simulink model "Final_Cloud"  (R2026a)
settings: Solver=FixedStepAuto  StopTime=inf  FixedStep=0.01  EnableMultiTasking=on
undefined symbols (not defined in the file or in its folder): Kg, Kt, r, R_m, V_batt
libraries: arduinolib x7, arduinosensorlib x1, slpidlib x1
settings Model: SimulationMode=external  SILPILModeSetting=veronly  ExtModeTrigDuration=2  Creator=Adham  LastModifiedBy=Adham
settings HardwareCC: ProdLargestAtomicInteger=Long  ProdLargestAtomicFloat=Double  ProdHWDeviceType=ARM Compatible->ARM Cortex  UseEmbeddedCoderFeatures=off
settings RTWCC: SystemTargetFile=ert.tlc  HardwareBoard=ESP32-WROOM (Arduino Compatible)  TLCOptions="-aInlineSetEventsForThisBaseRateFcn=TLC_FALSE -aSuppressMultiTaskScheduler=TLC_FALSE  -aRateBasedStepFcn=0"  Toolchain=ESP32  BuildConfiguration=Faster Runs  Description=Embedded Coder
settings RTWCC: CustomInclude=|
  | C:\ProgramData\MATLAB\SupportPackages\R2026a\aCLI\data\packages\esp32\hardware\esp32\2.0.17\libraries\Wire\src
  | D:\CoTune2026\Active_Suspension_resources\Parameter_Estimation_DAQ
  | D:\CoTune2026\Active_Suspension_resources\Parameter_Estimation_DAQ\core\inc
  | D:\CoTune2026\Active_Suspension_resources\Parameter_Estimation_DAQ\core\src
  | D:\CoTune2026\Active_Suspension_resources\Parameter_Estimation_DAQ\platform\inc
  | D:\CoTune2026\Active_Suspension_resources\Parameter_Estimation_DAQ\platform\src
  | C:\ProgramData\MATLAB\SupportPackages\R2026a\aCLI\data\packages\esp32\hardware\esp32\2.0.17\libraries\WiFi\src
  | C:\ProgramData\MATLAB\SupportPackages\R2026a\aCLI\data\packages\esp32\hardware\esp32\2.0.17\libraries\WiFiClientSecure\src
  | C:\Users\Dell\Documents\Arduino\libraries\PubSubClient\src
  | C:\Users\Dell\Documents\Arduino\libraries\ArduinoJson\src
settings RTWCC: CustomSource=|
  | C:\ProgramData\MATLAB\SupportPackages\R2026a\aCLI\data\packages\esp32\hardware\esp32\2.0.17\libraries\Wire\src\Wire.cpp
  | core\src\vl53l0x_api.cpp
  | core\src\vl53l0x_api_calibration.cpp
  | core\src\vl53l0x_api_core.cpp
  | core\src\vl53l0x_api_ranging.cpp
  | core\src\vl53l0x_api_strings.cpp
  | platform\src\vl53l0x_platform.cpp
  | Adafruit_VL53L0X.cpp
  | C:\Users\Dell\Documents\Arduino\libraries\PubSubClient\src\PubSubClient.cpp
  | C:\ProgramData\MATLAB\SupportPackages\R2026a\aCLI\data\packages\esp32\hardware\esp32\2.0.17\libraries\WiFi\src\WiFi.cpp
  | C:\ProgramData\MATLAB\SupportPackages\R2026a\aCLI\data\packages\esp32\hardware\esp32\2.0.17\libraries\WiFi\src\WiFiSTA.cpp
  | C:\ProgramData\MATLAB\SupportPackages\R2026a\aCLI\data\packages\esp32\hardware\esp32\2.0.17\libraries\WiFi\src\WiFiGeneric.cpp
  | C:\ProgramData\MATLAB\SupportPackages\R2026a\aCLI\data\packages\esp32\hardware\esp32\2.0.17\libraries\WiFi\src\WiFiClient.cpp
  | C:\ProgramData\MATLAB\SupportPackages\R2026a\aCLI\data\packages\esp32\hardware\esp32\2.0.17\libraries\WiFiClientSecure\src\WiFiClientSecure.cpp
  | C:\ProgramData\MATLAB\SupportPackages\R2026a\aCLI\data\packages\esp32\hardware\esp32\2.0.17\libraries\WiFiClientSecure\src\ssl_client.cpp
  | C:\ProgramData\MATLAB\SupportPackages\R2026a\aCLI\data\packages\esp32\hardware\esp32\2.0.17\libraries\WiFi\src\WiFiScan.cpp
  | C:\ProgramData\MATLAB\SupportPackages\R2026a\aCLI\data\packages\esp32\hardware\esp32\2.0.17\libraries\WiFi\src\WiFiAP.cpp
  | C:\ProgramData\MATLAB\SupportPackages\R2026a\aCLI\data\packages\esp32\hardware\esp32\2.0.17\libraries\WiFi\src\WiFiUdp.cpp
settings ERTTargetCC: ExtModeTransport=3.0  ExtModeAutomaticAllocSize=off  ExtModeStaticAllocSize=65536.0  SupportContinuousTime=on  SupportNonInlinedSFcns=on  SupportVariableSizeSignals=on

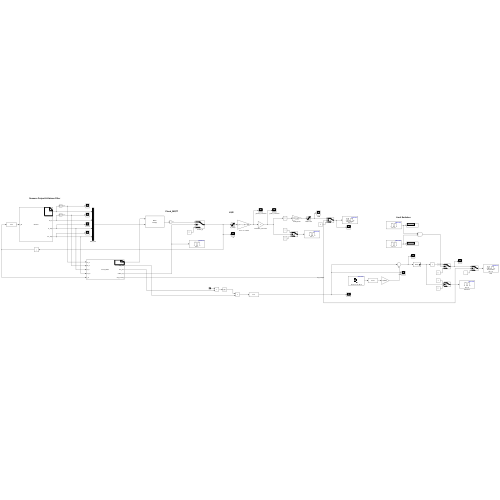
[thumbnail: Simulink's stored preview of the top-level diagram]
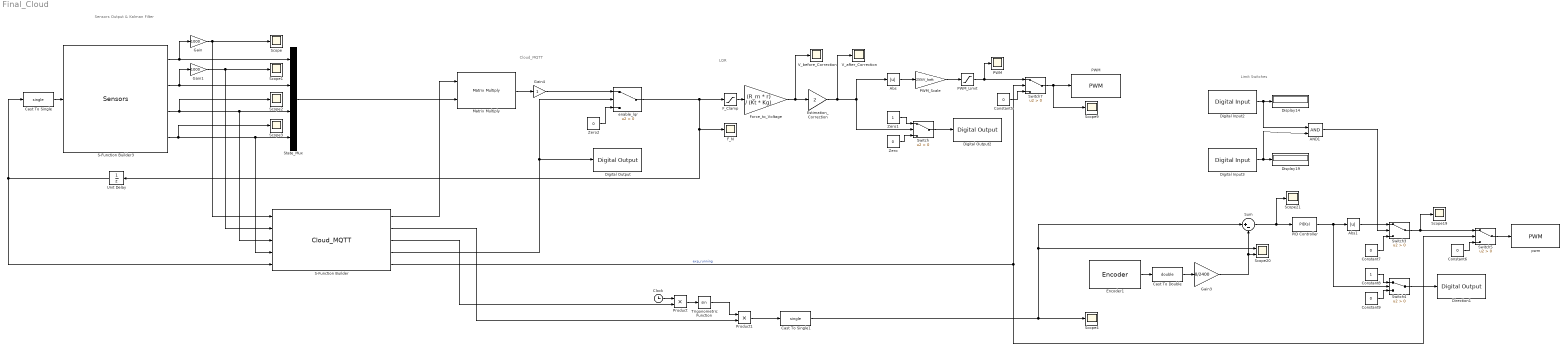
== system Final_Cloud ==
  note: Limit Switches
  note: Sensors Output & Kalman Filter
  note: LQR
  note: Cloud_MQTT
  AND1 : Logic  IconShape=distinctive  AllPortsSameDT=off  OutDataTypeStr=boolean
  Abs : Abs  SaturateOnIntegerOverflow=off
  Abs1 : Abs  SaturateOnIntegerOverflow=off
  Cast To Double : DataTypeConversion  OutDataTypeStr=double  SaturateOnIntegerOverflow=off  RndMeth=Floor
  Cast To Single : DataTypeConversion  OutDataTypeStr=single  SaturateOnIntegerOverflow=off  RndMeth=Floor
  Cast To Single1 : DataTypeConversion  OutDataTypeStr=single  SaturateOnIntegerOverflow=off  RndMeth=Floor
  Clock : Clock
  Constant{5..7,9} (4 alike) : Constant  Value=0
  Constant8 : Constant
  Digital Input2 : arduinolib/Digital Input  pinNumber=16  mode=Input Pullup  Direction=input  SampleTime=0.1  blockPlatform=arduino
  Digital Input3 : arduinolib/Digital Input  pinNumber=17  mode=Input Pullup  Direction=input  SampleTime=0.1  blockPlatform=arduino
  Digital Output : arduinolib/Digital Output  pinNumber=2  Direction=output  blockPlatform=arduino
  Digital Output2 : arduinolib/Digital Output  pinNumber=4  Direction=output  blockPlatform=arduino
  Direction1 : arduinolib/Digital Output  pinNumber=18  Direction=output  blockPlatform=arduino
  Display14 : Display
  Display19 : Display
  Encoder1 : arduinosensorlib/Encoder  InputA=13  InputB=14  Mode=No reset  SampleTime=-1
  Estimation_Correction : Gain  Gain=2
  F_Clamp : Saturate  UpperLimit=10  LowerLimit=-10
  F_N : Scope
      settings: ActiveDisplayYMinimum=-32.354349136352539  ActiveDisplayYMaximum=27.611242294311523  DataLoggingVariableName=ScopeData5
  Force_to_Voltage : Gain  Gain=(R_m * r) / (Kt * Kg)
  Gain : Gain  Gain=1000
  Gain1 : Gain  Gain=1000
  Gain3 : Gain  Gain=8/2400
  Gain4 : Gain
  Matrix Multiply : Product  Multiplication=Matrix(*)
  PID Controller : slpidlib/PID Controller  Controller=PID  Form=Parallel  TimeDomain=Continuous-time  UseExternalTs=off  SampleTime=-1  IntegratorMethod=Forward Euler  FilterMethod=Forward Euler  ControllerParametersSource=internal  P=20  I=0  UseKiTs=off  D=0  UseExternalDerivativeSource=off  N=100  UseFilter=on  TunerSelectOption=Transfer Function Based (PID Tuner App)  InitialConditionSource=internal  InitialConditionForIntegrator=0  InitialConditionForFilter=0  DifferentiatorICPrevScaledInput=0  ExternalReset=none  TrackingMode=off  Kt=1  LimitOutput=on  SatLimitsSource=internal  UpperSaturationLimit=255  LowerSaturationLimit=-255  LinearizeAsGain=on  AntiWindupMode=none  Kb=1  LimitIntegrator=off  UpperIntegratorSaturationLimit=inf  LowerIntegratorSaturationLimit=-inf  POutMin=[]  POutMax=[]  IOutMin=[]  IOutMax=[]  DOutMin=[]  DOutMax=[]  NOutMin=[]  NOutMax=[]  SumOutMin=[]  SumOutMax=[]  SaturationOutMin=[]  SaturationOutMax=[]  PParamMin=[]  PParamMax=[]  IParamMin=[]  IParamMax=[]  DParamMin=[]  DParamMax=[]  NParamMin=[]  NParamMax=[]  KbParamMin=[]  KbParamMax=[]  KtParamMin=[]  KtParamMax=[]  KbOutMin=[]  KbOutMax=[]  KtOutMin=[]  KtOutMax=[]  IntegratorOutMin=[]  IntegratorOutMax=[]  FilterOutMin=[]  FilterOutMax=[]  SumI1OutMin=[]  SumI1OutMax=[]  SumI2OutMin=[]  SumI2OutMax=[]  SumI3OutMin=[]  SumI3OutMax=[]  SumI4OutMin=[]  SumI4OutMax=[]  SumDOutMin=[]  SumDOutMax=[]  DifferentiatorOutMin=[]  DifferentiatorOutMax=[]  FilterDiffOutCoefMin=[]  FilterDiffOutCoefMax=[]  ReciprocalOutMin=[]  ReciprocalOutMax=[]  SumDenOutMin=[]  SumDenOutMax=[]  SumNumOutMin=[]  SumNumOutMax=[]  DivideOutMin=[]  DivideOutMax=[]  UdiffTsProdOutMin=[]  UdiffTsProdOutMax=[]  NTsProdOutMin=[]  NTsProdOutMax=[]  UintegralTsProdOutMin=[]  UintegralTsProdOutMax=[]  UngainTsProdOutMin=[]  UngainTsProdOutMax=[]  ClampingZeroOutDataTypeStr=Inherit: Inherit via back propagation  ClampingZeroOutMin=[]  ClampingZeroOutMax=[]  FilterDenConstantOutDataTypeStr=Inherit: Inherit via back propagation  FilterDenConstantOutMin=[]  FilterDenConstantOutMax=[]  PCopyOutDataTypeStr=Inherit: Inherit via back propagation  PCopyOutMin=[]  PCopyOutMax=[]  NCopyOutDataTypeStr=Inherit: Inherit via back propagation  NCopyOutMin=[]  NCopyOutMax=[]  IntegratorContinuousStateAttributes=''  IntegratorStateMustResolveToSignalObject=off  IntegratorRTWStateStorageClass=Auto  FilterContinuousStateAttributes=''  FilterStateMustResolveToSignalObject=off  FilterRTWStateStorageClass=Auto  ParallelPVariant=InternalParameters  IdealPVariant=Disabled  IVariant=InternalParameters  DVariant=InternalParameters  IntegratorVariant=Continuous  SatVariant=Enabled  AWVariant=Passthrough  PCopyVariant=Disabled  TRVariant=Disabled  FdbkBlocksVariant=Forward  IdealPFdbkVariant=Disabled  SatFdbkVariant=Disabled  DerivativeFilterVariant=ContFilter  NVariant=InternalParameters  NCopyVariant=Disabled  FilterICVariant=InternalICsFilter  IntegratorICVariant=InternalICs  ExternalResetVariant=Disabled  TRSumVariant=Passthrough  SumFdbkVariant=Disabled  SumVariant=Sum_PID  TsampFilterVariant=InternalTs  TsampNgainVariant=Passthrough  TsampIntegralVariant=Disabled_SignalSpec  ExternalSaturationOutDataTypeStr=Inherit: Same as second input  DerivativeSourceVariant=ErrorSignal  PreIntVariant=InternalPreInt
  PWM : arduinolib/PWM  pinNumber=5  frequencyType=Default  desiredFrequency=490.2  achievableFrequency=490.2
  "PWM " : Scope
      settings: ActiveDisplayYMinimum=-4.2180590409916467  ActiveDisplayYMaximum=37.966469179467822  DataLoggingVariableName=ScopeData7
  PWM_Limit : Saturate  UpperLimit=255  LowerLimit=0
  PWM_Scale : Gain  Gain=255/V_batt
  Product : Product
  Product1 : Product
  S-Function Builder : S-Function  FunctionName=Cloud_MQTT  SFunctionModules=Cloud_MQTT_wrapper.cpp  SFunctionDeploymentMode=off  EnableBusSupport=off  mask(S-Function Builder){}
      mask help: Simulink:masks:SFunctionBuilder_MD
      mask init:
      | val = [[.9  0.75 0.75 1 1 .9 .9 1]',[1 1 0.75 0.75 .9 .9 1 .9]'];try , sys = get_param(gcb,'SfunBuilderFcnName');if isempty(sys), sys = get_param(gcb,'FunctionName'); end,catch, sys = get_param(gcb,'FunctionName'); end
      settings: CopyFcn=set_param(gcbh,'LinkStatus','none')  OpenFcn=sfunctionwizard(gcbh)
      mask Display:
      | plot(val(:,1),val(:,2))
      | disp(sys)
      | port_label('input',1,sprintf('%s', 'd1\_in'),'interpreter','tex')
      | port_label('input',2,sprintf('%s', 'd2\_in'),'interpreter','tex')
      | port_label('input',3,sprintf('%s', 'vs\_in'),'interpreter','tex')
      | port_label('input',4,sprintf('%s', 'vus\_in'),'interpreter','tex')
      | port_label('input',5,sprintf('%s', 'u\_in'),'interpreter','tex')
      | port_label('output',1,sprintf('%s', 'K\_out'),'interpreter','tex')
      | port_label('output',2,sprintf('%s', 'amp\_out'),'interpreter','tex')
      | port_label('output',3,sprintf('%s', 'freq\_out'),'interpreter','tex')
      | port_label('output',4,sprintf('%s', 'enable\_lqr'),'interpreter','tex')
      | port_label('output',5,sprintf('%s', 'exp\_running'),'interpreter','tex')
  S-Function Builder3 : S-Function  FunctionName=Sensors  SFunctionModules=Sensors_wrapper.cpp  SFunctionDeploymentMode=off  EnableBusSupport=off  mask(S-Function Builder){}
      mask help: Simulink:masks:SFunctionBuilder_MD
      mask init: same as Final_Cloud/S-Function Builder
      settings: CopyFcn=set_param(gcbh,'LinkStatus','none')  OpenFcn=sfunctionwizard(gcbh)
      mask Display:
      | plot(val(:,1),val(:,2))
      | disp(sys)
      | port_label('input',1,sprintf('%s', 'u\_N'),'interpreter','tex')
      | port_label('output',1,sprintf('%s', 'd1\_m'),'interpreter','tex')
      | port_label('output',2,sprintf('%s', 'd2\_m'),'interpreter','tex')
      | port_label('output',3,sprintf('%s', 'vs\_mps'),'interpreter','tex')
      | port_label('output',4,sprintf('%s', 'vus\_mps'),'interpreter','tex')
  Scope{,1..4,9,19,21} (8 alike) : Scope
      Scope settings: ActiveDisplayYMinimum=-23.180127382278442  ActiveDisplayYMaximum=14.85132908821106
      Scope1 settings: ActiveDisplayYMinimum=-10.222212970256805  ActiveDisplayYMaximum=15.830363929271698
      Scope19 settings: ActiveDisplayYMinimum=-19.129211768390523  ActiveDisplayYMaximum=172.16290591551473  DataLoggingVariableName=ScopeData21
      Scope2 settings: ActiveDisplayYMinimum=-0.27071841806173325  ActiveDisplayYMaximum=0.26262833923101425  DataLoggingVariableName=ScopeData2
      Scope21 settings: ActiveDisplayYMinimum=-49.886250000000004  ActiveDisplayYMaximum=49.54291666666667  DataLoggingVariableName=ScopeData23
      Scope3 settings: ActiveDisplayYMinimum=-0.35517418943345547  ActiveDisplayYMaximum=0.24406235478818417  DataLoggingVariableName=ScopeData3
      Scope4 settings: ActiveDisplayYMinimum=-49.886250000000004  ActiveDisplayYMaximum=49.54291666666667  DataLoggingVariableName=ScopeData8
      Scope9 settings: ActiveDisplayYMinimum=-12.6555061340332  ActiveDisplayYMaximum=113.89955520629883  DataLoggingVariableName=ScopeData9
  Scope20 : Scope  NumInputPorts=2
      settings: ActiveDisplayYMinimum=-18.854999982749238  ActiveDisplayYMaximum=19.694999998083247  DataLoggingVariableName=ScopeData22
  State_Mux : Mux
  Sum : Sum  Inputs=|+-
  Switch{,3..5,7} (5 alike) : Switch  Criteria=u2 > Threshold  SaturateOnIntegerOverflow=off  InputSameDT=off
  Trigonometric Function : Trigonometry
  Unit Delay : UnitDelay  SampleTime=-1
  V_after_Correction : Scope
      settings: ActiveDisplayYMinimum=-3.9703547954559326  ActiveDisplayYMaximum=3.9703547954559326  DataLoggingVariableName=ScopeData6
  V_before_Correction : Scope
      settings: ActiveDisplayYMinimum=-1.9851773977279663  ActiveDisplayYMaximum=1.9851773977279663  DataLoggingVariableName=ScopeData4
  Zero : Constant  Value=0
  Zero1 : Constant
  Zero2 : Constant  Value=0  OutDataTypeStr=Inherit: Inherit via back propagation
  enable_lqr : Switch  Criteria=u2 > Threshold  SaturateOnIntegerOverflow=off  InputSameDT=off
  pwm : arduinolib/PWM  pinNumber=19  frequencyType=Default  desiredFrequency=490.2  achievableFrequency=490.2
  wires:
  Digital Input3/1 -> AND1/2, Display19/1
  AND1/1 -> Switch3/2
  Constant7/1 -> Switch3/3
  Switch3/1 -> Scope19/1, Switch5/1
  Switch4/1 -> Direction1/1
  Constant9/1 -> Switch4/3
  Constant8/1 -> Switch4/1
  Sum/1 -> PID Controller/1, Scope21/1
  Digital Input2/1 -> AND1/1, Display14/1
  Gain3/1 -> Sum/2, Scope20/2
  PID Controller/1 -> Switch4/2, Abs1/1
  S-Function Builder/5 -> Switch5/2, Switch7/2  "exp_running"
  Constant6/1 -> Switch5/3
  Switch5/1 -> pwm/1
  Encoder1/1 -> Cast To Double/1
  Cast To Double/1 -> Gain3/1
  Zero1/1 -> Switch/1
  Switch/1 -> Digital Output2/1
  PWM_Scale/1 -> PWM_Limit/1
  Abs/1 -> PWM_Scale/1
  Force_to_Voltage/1 -> V_before_Correction/1, Estimation_Correction/1
  PWM_Limit/1 -> "PWM "/1, Switch7/1
  State_Mux/1 -> Matrix Multiply/2
  Zero/1 -> Switch/3
  Switch7/1 -> PWM/1, Scope9/1
  Constant5/1 -> Switch7/3
  Product1/1 -> Cast To Single1/1
  enable_lqr/1 -> Unit Delay/1, F_N/1, F_Clamp/1
  Cast To Single/1 -> S-Function Builder3/1
  Gain/1 -> Scope/1, S-Function Builder/1
  Gain1/1 -> Scope1/1, S-Function Builder/2
  S-Function Builder3/3 -> State_Mux/3, S-Function Builder/3, Scope2/1
  S-Function Builder3/4 -> State_Mux/4, S-Function Builder/4, Scope3/1
  S-Function Builder3/1 -> State_Mux/1, Gain/1
  S-Function Builder3/2 -> State_Mux/2, Gain1/1
  F_Clamp/1 -> Force_to_Voltage/1
  Unit Delay/1 -> S-Function Builder/5, Cast To Single/1
  Estimation_Correction/1 -> Abs/1, Switch/2, V_after_Correction/1
  Abs1/1 -> Switch3/1
  S-Function Builder/1 -> Matrix Multiply/1
  Matrix Multiply/1 -> Gain4/1
  S-Function Builder/2 -> Product1/2
  S-Function Builder/3 -> Product/2
  Zero2/1 -> enable_lqr/3
  Gain4/1 -> enable_lqr/1
  S-Function Builder/4 -> Digital Output/1, enable_lqr/2
  Clock/1 -> Product/1
  Product/1 -> Trigonometric Function/1
  Trigonometric Function/1 -> Product1/1
  Cast To Single1/1 -> Scope20/1, Sum/1, Scope4/1
